simulink model "BOOST"  (R2023a)
settings: Solver=VariableStepAuto  StartTime=0.0  StopTime=0.01  RelTol=1e-3
libraries: spsCurrentMeasurementLib x3, spsVoltageMeasurementLib x3, spsSeriesRLCBranchLib x3, spsDCVoltageSourceLib x1, spsDiodeLib x1, spsMosfetLib x1, sps_lib x1
settings Model: Creator=prish  LastModifiedBy=prish

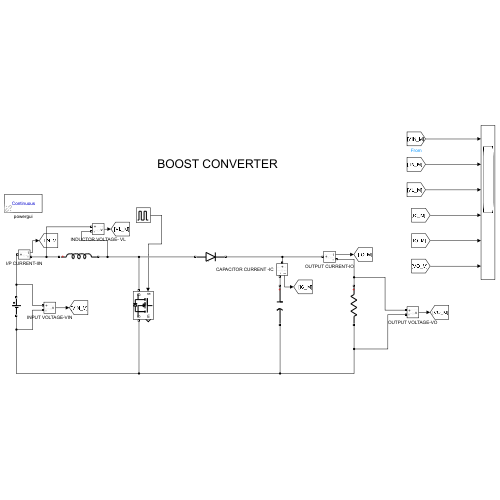
[thumbnail: Simulink's stored preview of the top-level diagram]
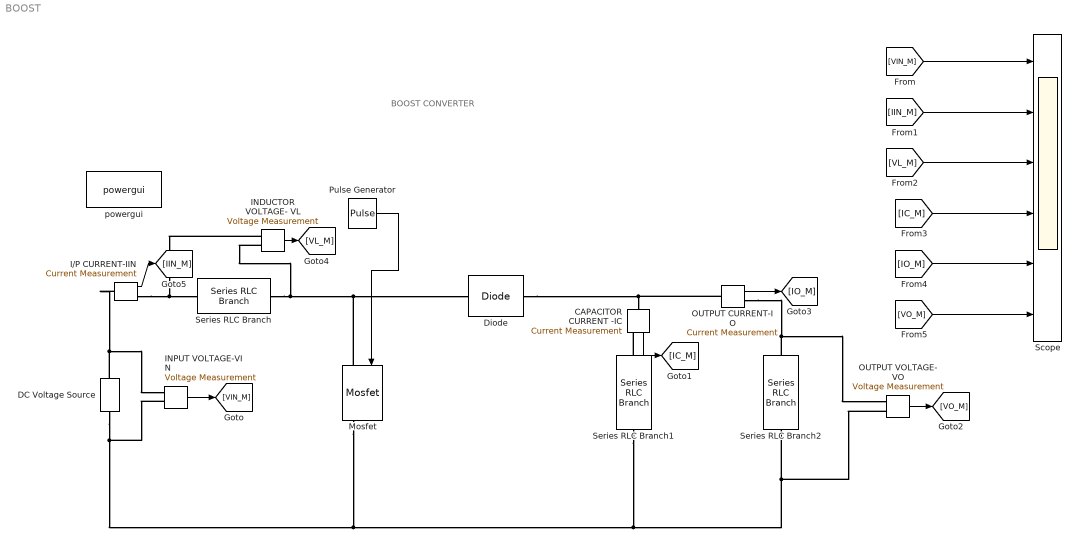
== system BOOST ==
  note: BOOST CONVERTER
  CAPACITOR CURRENT -IC : spsCurrentMeasurementLib/Current Measurement  PhasorSimulation=off  OutputType=Complex  PSBequivalent=0
  DC Voltage Source : spsDCVoltageSourceLib/DC Voltage Source  Amplitude=24  Measurements=None
  Diode : spsDiodeLib/Diode  Ron=0.001  Lon=0  Vf=0  IC=0  UseSnubber=0  Rs=inf  Cs=inf  Measurements=off
  I/P CURRENT-IIN : spsCurrentMeasurementLib/Current Measurement  PhasorSimulation=off  OutputType=Complex  PSBequivalent=0
  INDUCTOR VOLTAGE- VL : spsVoltageMeasurementLib/Voltage Measurement  PhasorSimulation=off  OutputType=Complex  PSBequivalent=0
  INPUT VOLTAGE-VIN : spsVoltageMeasurementLib/Voltage Measurement  PhasorSimulation=off  OutputType=Complex  PSBequivalent=0
  Mosfet : spsMosfetLib/Mosfet  Ron=1e-3  Lon=0  Rd=1e-3  Vfd=0  IC=0  Rs=1e5  Cs=inf  Measurements=on
  OUTPUT CURRENT-IO : spsCurrentMeasurementLib/Current Measurement  PhasorSimulation=off  OutputType=Complex  PSBequivalent=0
  OUTPUT VOLTAGE-VO : spsVoltageMeasurementLib/Voltage Measurement  PhasorSimulation=off  OutputType=Complex  PSBequivalent=0
  Pulse Generator : DiscretePulseGenerator  PulseType=Time based  Period=10  PulseWidth=5
  Scope : Scope  NumInputPorts=6
  Series RLC Branch : spsSeriesRLCBranchLib/Series RLC Branch  LConnTagsString=__new0  RConnTagsString=__new0  BranchType=L  Resistance=1e-3  Inductance=250e-6  SetiL0=off  InitialCurrent=0  Capacitance=1e-6  Setx0=off  InitialVoltage=0  Measurements=None
  Series RLC Branch1 : spsSeriesRLCBranchLib/Series RLC Branch  LConnTagsString=__new0  RConnTagsString=__new0  BranchType=C  Resistance=1  Inductance=1e-3  SetiL0=off  InitialCurrent=0  Capacitance=200e-6  Setx0=off  InitialVoltage=0  Measurements=None
  Series RLC Branch2 : spsSeriesRLCBranchLib/Series RLC Branch  LConnTagsString=__new0  RConnTagsString=__new0  BranchType=R  Resistance=3  Inductance=1e-3  SetiL0=off  InitialCurrent=0  Capacitance=1e-6  Setx0=off  InitialVoltage=0  Measurements=None
  powergui : sps_lib/powergui  Priority=1  SimulationMode=Continuous  SampleTime=50e-6  frequency=60  Iterations=50  frequencyindice=0  Pbase=100e6  ErrMax=1e-4  UnitsV=kV  UnitsW=MW  buscounter=0  FunctionMessages=off  echomessages=off  EnableUseOfTLC=off  CurrentSourceSwitches=off  DisableSnubberDevices=off  DisableRonSwitches=off  DisableVfSwitches=off  DisplayEquations=off  AutomaticDiscreteSolvers=off  SolverType=Tustin/Backward Euler (TBE)  Interpol=off  ExternalGateDelay=off  methode=off  Ts=100  x0status=blocks  SPID=on  SwTol=0  HookPort=off  NonlinearTolerance=1e-4  nMaxIteration=100  ContinueOnMaxIteration=off  RestoreLinks=warning  ResistiveCurrentMeasurement=off  Frange=[0:2:500]  Ylog=off  Xlog=on  ShowGrid=off  save=off  variable=ZData  structure=0  ZoomFFT=off  StartTime=0.0  cycles=1  DisplayStyle=1  fundamental=60  FreqAxis=off  MaxFrequency=1000  frequencyindicesteady=1  RmsSteady=1  display=off
  wires:
  Pulse Generator/1 -> Mosfet/1
  INPUT VOLTAGE-VIN/1 -> [VIN_M]
  INDUCTOR VOLTAGE- VL/1 -> [VL_M]
  OUTPUT CURRENT-IO/1 -> [IO_M]
  OUTPUT VOLTAGE-VO/1 -> [VO_M]
  CAPACITOR CURRENT -IC/1 -> [IC_M]
  I/P CURRENT-IIN/1 -> [IIN_M]
  [VO_M] -> Scope/6
  [IC_M] -> Scope/4
  [IO_M] -> Scope/5
  [VIN_M] -> Scope/1
  [VL_M] -> Scope/3
  [IIN_M] -> Scope/2
  connections:
  INDUCTOR VOLTAGE- VL/LConn1 -- Series RLC Branch/LConn1 -- I/P CURRENT-IIN/RConn1
  Series RLC Branch/RConn1 -- INDUCTOR VOLTAGE- VL/LConn2 -- Mosfet/LConn1 -- Diode/LConn1
  DC Voltage Source/LConn1 -- INPUT VOLTAGE-VIN/LConn2 -- Mosfet/RConn1 -- OUTPUT VOLTAGE-VO/LConn2 -- Series RLC Branch2/RConn1 -- Series RLC Branch1/RConn1
  Diode/RConn1 -- OUTPUT CURRENT-IO/LConn1 -- CAPACITOR CURRENT -IC/LConn1
  Series RLC Branch1/LConn1 -- CAPACITOR CURRENT -IC/RConn1
  DC Voltage Source/RConn1 -- I/P CURRENT-IIN/LConn1 -- INPUT VOLTAGE-VIN/LConn1
  Series RLC Branch2/LConn1 -- OUTPUT CURRENT-IO/RConn1 -- OUTPUT VOLTAGE-VO/LConn1
